simulink model "Simulacao_3C"  (R2015a)
settings: Solver=ode45  StartTime=0.0  StopTime=240  FixedStep=0.1  MaxStep=5e-1  RelTol=1e-3
values from neighbouring files (symbols this model uses):
  A = [-(a1/A1)*sqrt(g/(2*L10)) 0 ... (first row only)    [calc_sd_oe.m]
  B = [Km/A1; 0]    [calc_sd_oe.m]
  C = [0 1]    [calc_sd_oe.m]
  K1 = real(Ka(1))    [calc_sd_oe.m]
  K2 = real([Ka(2) Ka(3)])    [calc_sd_oe.m]
  L = qlA*inv(V)*[0;1]    [calc_sd_oe.m]
libraries: simulink x6
settings Model: CovSFcnEnable=off  Creator=MeneghettiAir  LastModifiedBy=hemerson
settings DebuggingCC: SolverPrmCheckMsg=warning

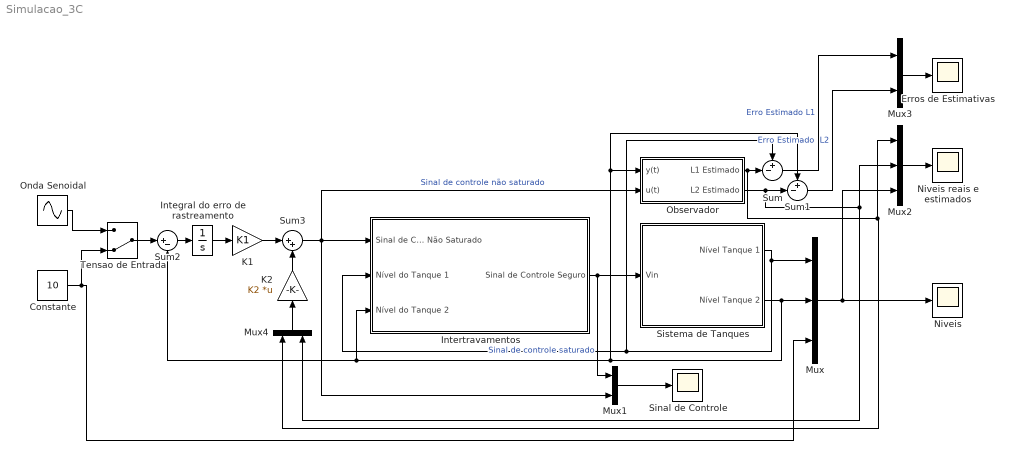
== system Simulacao_3C ==
  Constante : Constant  Value=10
  Erros de Estimativas : Scope
      settings: ShowLegends=on  TimeRange=240  YMax=35  SaveName=Niveis2  MaxDataPoints=500000
  Integral do erro de rastreamento : Integrator
  Intertravamentos : Subsystem
  K1 : Gain  Gain=K1
  K2 : Gain  Gain=K2  Multiplication=Matrix(K*u)
  Mux : Mux  Inputs=3
  Mux1 : Mux  Inputs=2
  Mux2 : Mux  Inputs=3
  Mux3 : Mux  Inputs=2
  Mux4 : Mux  Inputs=2
  Niveis : Scope
      settings: ShowLegends=on  TimeRange=240  YMin=5  YMax=30  SaveName=Niveis  MaxDataPoints=500000
  Niveis reais e estimados : Scope
      settings: ShowLegends=on  TimeRange=240  YMin=5  YMax=32.5  SaveName=Niveis1  MaxDataPoints=500000
  Observador : Subsystem
  Onda Senoidal : Sin  Amplitude=2  Bias=2  Frequency=0.2  SampleTime=0
  Sinal de Controle : Scope
      settings: ShowLegends=on  TimeRange=240  YMin=-1  YMax=6  MaxDataPoints=500000
  "Sistema de Tanques " : Subsystem
  Sum : Sum  Inputs=+-|
  Sum1 : Sum  Inputs=+-|
  Sum2 : Sum  Inputs=|+-
  Sum3 : Sum  Inputs=|++
  Tensao de Entrada : ManualSwitch  CurrentSetting=0
  wires:
  Mux/1 -> Mux2/3, Niveis/1
  Constante/1 -> Mux/3, Tensao de Entrada/2
  Onda Senoidal/1 -> Tensao de Entrada/1
  "Sistema de Tanques "/1(Nível Tanque 1) -> Intertravamentos/2(Nível do Tanque 1), Sum/1, Mux/1
  "Sistema de Tanques "/2(Nível Tanque 2) -> Mux/2, Sum2/2, Intertravamentos/3(Nível do Tanque 2), Sum1/1, Observador/1(y(t))
  Mux2/1 -> Niveis reais e estimados/1
  Sum/1 -> Mux3/1  "Erro Estimado L1"
  Mux3/1 -> Erros de Estimativas/1
  Sum1/1 -> Mux3/2  "Erro Estimado  L2"
  Observador/2(L2 Estimado) -> Mux2/2, Mux4/2, Sum1/2
  Tensao de Entrada/1 -> Sum2/1
  Intertravamentos/1(Sinal de Controle Seguro) -> Mux1/1, "Sistema de Tanques "/1(Vin)  "Sinal de controle saturado"
  Integral do erro de rastreamento/1 -> K1/1
  K1/1 -> Sum3/1
  Sum2/1 -> Integral do erro de rastreamento/1
  Sum3/1 -> Observador/2(u(t)), Mux1/2, Intertravamentos/1(Sinal de Controle Não Saturado)  "Sinal de controle não saturado"
  Mux4/1 -> K2/1
  K2/1 -> Sum3/2
  Mux1/1 -> Sinal de Controle/1
  Observador/1(L1 Estimado) -> Mux2/1, Mux4/1, Sum/2

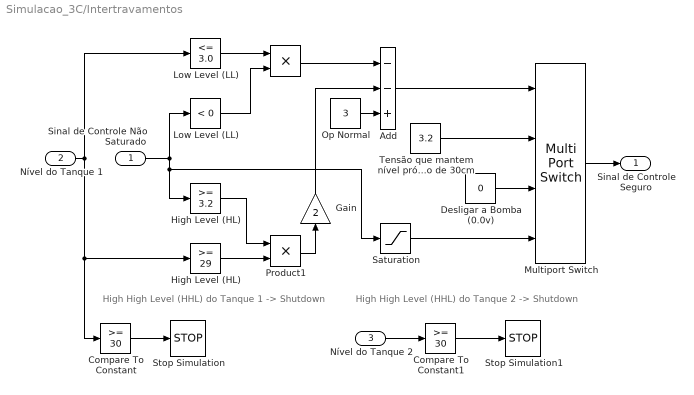
== system Simulacao_3C/Intertravamentos ==
  note: High High Level (HHL) do Tanque 1 -> Shutdown
  note: High High Level (HHL) do Tanque 2 -> Shutdown
  Sinal de Controle Não Saturado : Inport
  Nível do Tanque 1 : Inport  Port=2
  Nível do Tanque 2 : Inport  Port=3
  " " : Product
  " High Level (HL)" : simulink/Logic and Bit Operations/Compare To Constant  relop=>=  const=29  OutDataTypeStr=boolean
  " Low Level (LL) " : simulink/Logic and Bit Operations/Compare To Zero  relop=<  OutDataTypeStr=boolean
  Add : Sum  Inputs=--+
  Compare To Constant : simulink/Logic and Bit Operations/Compare To Constant  relop=>=  const=30  OutDataTypeStr=boolean
  Compare To Constant1 : simulink/Logic and Bit Operations/Compare To Constant  relop=>=  const=30  OutDataTypeStr=boolean
  Desligar a Bomba (0.0v) : Constant  Value=0
  Gain : Gain  Gain=2
  High Level (HL) : simulink/Logic and Bit Operations/Compare To Constant  relop=>=  const=3.2  OutDataTypeStr=boolean
  Low Level (LL) : simulink/Logic and Bit Operations/Compare To Constant  relop=<=  const=3.0  OutDataTypeStr=boolean
  Multiport Switch : MultiPortSwitch
  Op Normal : Constant  Value=3
  Product1 : Product
  Saturation : Saturate  UpperLimit=4  LowerLimit=-4
  Stop Simulation : Stop
  Stop Simulation1 : Stop
  Tensão que mantem nível próximo de 30cm : Constant  Value=3.2
  Sinal de Controle Seguro : Outport
  wires:
  Compare To Constant1/1 -> Stop Simulation1/1
  Nível do Tanque 2/1 -> Compare To Constant1/1
  Compare To Constant/1 -> Stop Simulation/1
  Nível do Tanque 1/1 -> Low Level (LL)/1, " High Level (HL)"/1, Compare To Constant/1
  Desligar a Bomba (0.0v)/1 -> Multiport Switch/3
  Tensão que mantem nível próximo de 30cm/1 -> Multiport Switch/2
  Add/1 -> Multiport Switch/1
  Op Normal/1 -> Add/3
  Gain/1 -> Add/2
  Product1/1 -> Gain/1
  " "/1 -> Add/1
  Sinal de Controle Não Saturado/1 -> Saturation/1, High Level (HL)/1, " Low Level (LL) "/1
  " Low Level (LL) "/1 -> " "/2
  Low Level (LL)/1 -> " "/1
  High Level (HL)/1 -> Product1/1
  " High Level (HL)"/1 -> Product1/2
  Multiport Switch/1 -> Sinal de Controle Seguro/1
  Saturation/1 -> Multiport Switch/4

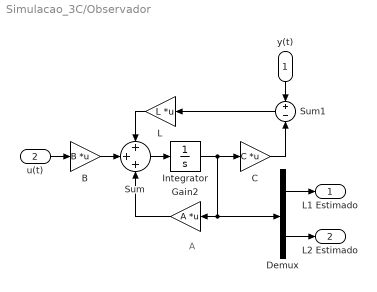
== system Simulacao_3C/Observador ==
  note: A
  y(t) : Inport
  u(t) : Inport  Port=2
  B : Gain  Gain=B  Multiplication=Matrix(K*u)
  C : Gain  Gain=C  Multiplication=Matrix(K*u)
  Demux : Demux  Outputs=2
  Gain2 : Gain  Gain=A  Multiplication=Matrix(K*u)
  Integrator : Integrator
  L : Gain  Gain=L  Multiplication=Matrix(K*u)
  Sum : Sum  Inputs=+++
  Sum1 : Sum  Inputs=+-
  L1 Estimado : Outport
  L2 Estimado : Outport  Port=2
  wires:
  u(t)/1 -> B/1
  B/1 -> Sum/2
  Gain2/1 -> Sum/3
  L/1 -> Sum/1
  Sum/1 -> Integrator/1
  Integrator/1 -> C/1, Demux/1, Gain2/1
  Sum1/1 -> L/1
  C/1 -> Sum1/2
  y(t)/1 -> Sum1/1
  Demux/2 -> L2 Estimado/1
  Demux/1 -> L1 Estimado/1

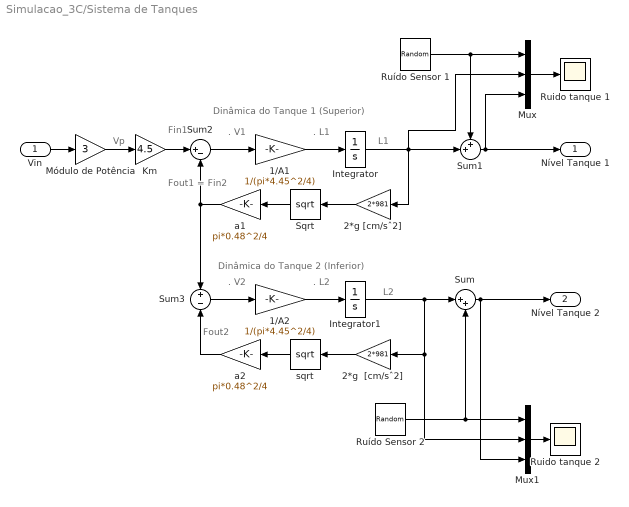
== system Simulacao_3C/Sistema de Tanques  ==
  note: Dinâmica do Tanque 1 (Superior)
  note: L1
  note: Fin1
  note: Fout1
      | =
      | Fin2
  note: .
      | L1
  note: .
      | V1
  note: L2
  note: Fout2
  note: .
      | L2
  note: .
      | V2
  note: Dinâmica do Tanque 2 (Inferior)
  note: Vp
  Vin : Inport
  1/A1 : Gain  Gain=1/(pi*4.45^2/4)
  1/A2 : Gain  Gain=1/(pi*4.45^2/4)
  2*g  [cm/sˆ2] : Gain  Gain=2*981
  2*g [cm/sˆ2] : Gain  Gain=2*981
  Integrator : Integrator  UpperSaturationLimit=35  LowerSaturationLimit=-2
  Integrator1 : Integrator  UpperSaturationLimit=35  LowerSaturationLimit=-2
  Km : Gain  Gain=4.5
  Mux : Mux  Inputs=3
  Mux1 : Mux  Inputs=3
  Módulo de Potência : Gain  Gain=3
  Ruido tanque 1 : Scope
      settings: TimeRange=50  YMin=0  YMax=20  SaveName=ScopeData3
  Ruido tanque 2 : Scope
      settings: TimeRange=50  YMin=0  YMax=20  SaveName=ScopeData4
  Ruído Sensor 1 : UniformRandomNumber  Minimum=-0.1  Maximum=0.1  Seed=round(rand(1)*100)  SampleTime=0.5
  Ruído Sensor 2 : UniformRandomNumber  Minimum=-0.1  Maximum=0.1  Seed=round(rand(1)*100)  SampleTime=0.7
  Sqrt : Sqrt  SaturateOnIntegerOverflow=on
  Sum : Sum  Inputs=|++
  Sum1 : Sum  Inputs=++|
  Sum2 : Sum  Inputs=|+-
  Sum3 : Sum  Inputs=+-
  a1 : Gain  Gain=pi*0.48^2/4
  a2 : Gain  Gain=pi*0.48^2/4
  sqrt : Sqrt  SaturateOnIntegerOverflow=on
  Nível Tanque 1 : Outport
  Nível Tanque 2 : Outport  Port=2
  wires:
  Vin/1 -> Módulo de Potência/1
  Sum/1 -> Nível Tanque 2/1, Mux1/3
  Mux/1 -> Ruido tanque 1/1
  Mux1/1 -> Ruido tanque 2/1
  Sum1/1 -> Nível Tanque 1/1, Mux/3
  Ruído Sensor 1/1 -> Mux/1, Sum1/1
  Ruído Sensor 2/1 -> Sum/2, Mux1/1
  2*g [cm/sˆ2]/1 -> Sqrt/1
  Sqrt/1 -> a1/1
  Km/1 -> Sum2/1
  a1/1 -> Sum2/2, Sum3/1
  Sum2/1 -> 1/A1/1
  1/A1/1 -> Integrator/1
  2*g  [cm/sˆ2]/1 -> sqrt/1
  sqrt/1 -> a2/1
  Sum3/1 -> 1/A2/1
  1/A2/1 -> Integrator1/1
  a2/1 -> Sum3/2
  Módulo de Potência/1 -> Km/1
  Integrator/1 -> Sum1/2, Mux/2, 2*g [cm/sˆ2]/1
  Integrator1/1 -> Mux1/2, 2*g  [cm/sˆ2]/1, Sum/1
